simulink model "Firstordercontrolsystem"  (Simulink 7.3)
settings: Solver=ode45  StartTime=0.0  StopTime=5.0  RelTol=1e-3
libraries: powerlib x1
settings Model: Creator=srija  LastModifiedBy=srija

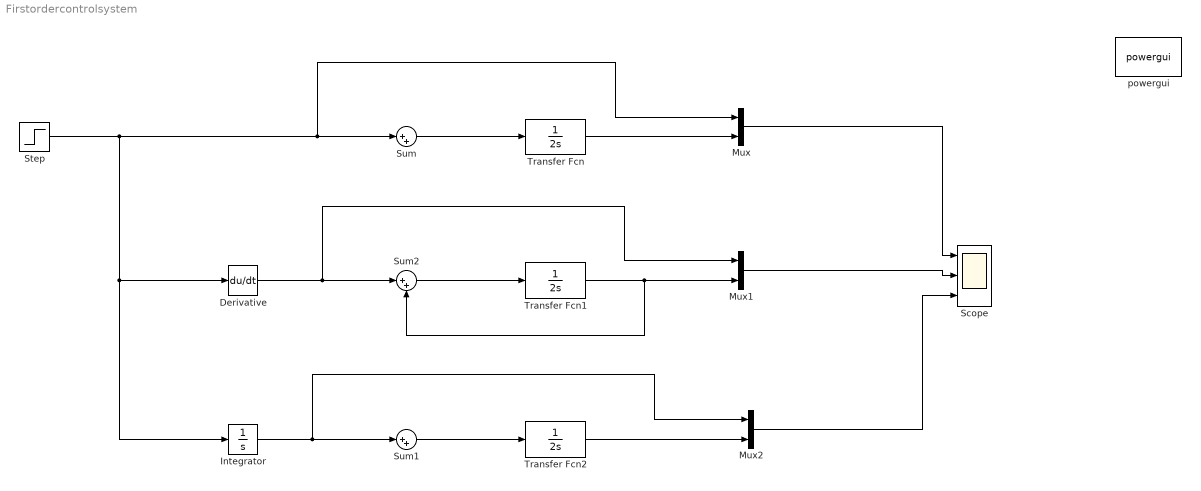
== system Firstordercontrolsystem ==
  Derivative : Derivative
  Integrator : Integrator
  Mux : Mux  Inputs=2
  Mux1 : Mux  Inputs=2
  Mux2 : Mux  Inputs=2
  Scope : Scope  NumInputPorts=3
      settings: YMin=-5~-5~-5  YMax=5~5~5
  Step : Step  After=100  SampleTime=0
  Sum : Sum  Inputs=|++  OutDataType=fixdt(1, 16)  OutScaling=2^0
  Sum1 : Sum  Inputs=|++  OutDataType=fixdt(1, 16)  OutScaling=2^0
  Sum2 : Sum  Inputs=|++  OutDataType=fixdt(1, 16)  OutScaling=2^0
  Transfer Fcn : TransferFcn  Denominator=[2 0]
  Transfer Fcn1 : TransferFcn  Denominator=[2 0]
  Transfer Fcn2 : TransferFcn  Denominator=[2 0]
  powergui : powerlib/powergui  Priority=1  SystemSampleTime=-1  SimulationMode=Continuous  SampleTime=50e-6  frequency=60  SPID=off  DisableSnubberDevices=off  DisableRonSwitches=off  DisableVfSwitches=off  SwTol=0  Interpol=off  frequencyindice=60  echomessages=off  HookPort=off  DisplayEquations=off  FunctionMessages=off  EnableUseOfTLC=off  x0status=blocks  RestoreLinks=warning  Frange=[0:2:500]  Ylog=off  Xlog=on  ShowGrid=off  save=off  variable=ZData  ZoomFFT=on  StartTime=0.0  cycles=1  DisplayStyle=1  fundamental=60  FreqAxis=off  MaxFrequency=1000  frequencyindicesteady=1  RmsSteady=1  display=off  Ts=0  methode=off
  wires:
  Sum/1 -> Transfer Fcn/1
  Step/1 -> Derivative/1, Integrator/1, Sum/1, Mux/1
  Integrator/1 -> Sum1/1, Mux2/1
  Derivative/1 -> Sum2/1, Mux1/1
  Sum2/1 -> Transfer Fcn1/1
  Sum1/1 -> Transfer Fcn2/1
  Transfer Fcn/1 -> Mux/2
  Transfer Fcn1/1 -> Mux1/2, Sum2/2
  Transfer Fcn2/1 -> Mux2/2
  Mux2/1 -> Scope/3
  Mux1/1 -> Scope/2
  Mux/1 -> Scope/1
